simulink library "NullCovarianceBus"  (R2018b)
settings: Solver=VariableStepAuto  StartTime=0.0  StopTime=10.0  RelTol=1e-3
settings Model: Creator=RA24876  LastModifiedBy=RA24876
settings SFSimCC: SimUseLocalCustomCode=off
settings RTWCC: RTWUseLocalCustomCode=off
settings CodeAppCC: StateflowObjectComments=on

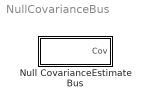
== system NullCovarianceBus ==
  Null CovarianceEstimate Bus : Subsystem  mask(Null CovarianceEstimate Bus){}
      mask help: Creates a CovarianceEstimate bus signal with all null values. Assign values to elements with a Bus Assignment block.

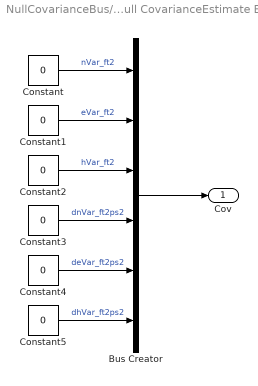
== system NullCovarianceBus/Null CovarianceEstimate Bus ==
  Bus Creator : BusCreator  Inputs=6  OutDataTypeStr=Bus: CovarianceEstimate
      settings: InheritFromInputs=off
  Constant{,1..5} (6 alike) : Constant  Value=0
  Cov : Outport  OutDataTypeStr=Bus: CovarianceEstimate
  wires:
  Constant2/1 -> Bus Creator/3  "hVar_ft2"
  Constant/1 -> Bus Creator/1  "nVar_ft2"
  Constant3/1 -> Bus Creator/4  "dnVar_ft2ps2"
  Constant5/1 -> Bus Creator/6  "dhVar_ft2ps2"
  Constant4/1 -> Bus Creator/5  "deVar_ft2ps2"
  Bus Creator/1 -> Cov/1
  Constant1/1 -> Bus Creator/2  "eVar_ft2"
